simulink model "HydroPowerSheet"  (R2017b)
settings: Solver=FixedStepDiscrete  StartTime=0.0  StopTime=365  FixedStep=1  RelTol=1e-3
undefined symbols (not defined in the file or in its folder): DiscIntNeverNeededParam
settings Model: Creator=h17163  LastModifiedBy=h17163

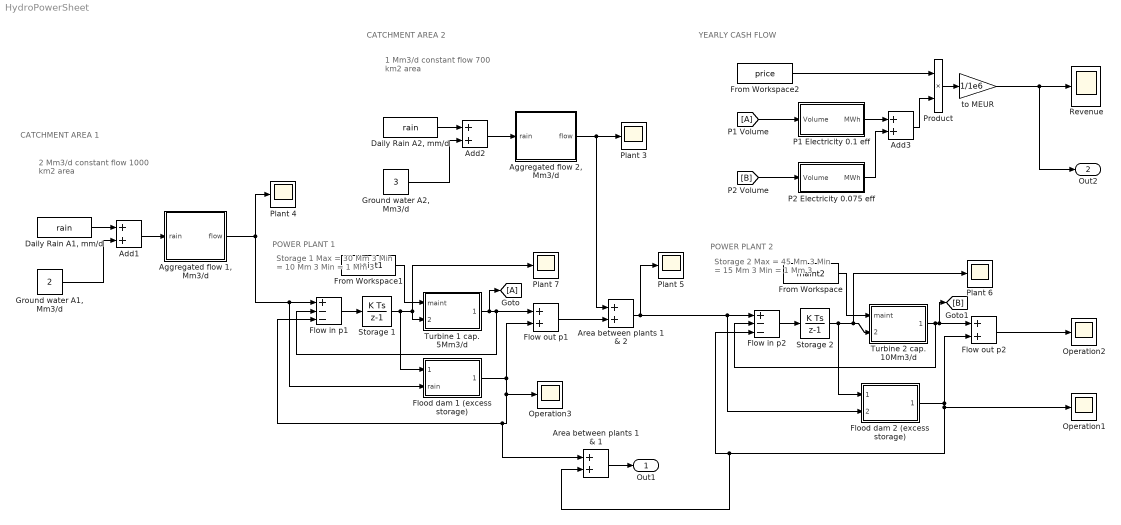
== system HydroPowerSheet ==
  note: YEARLY CASH FLOW
  note: 2 Mm3/d constant flow
      | 1000 km2 area
  note: POWER PLANT 1
  note: CATCHMENT AREA 1
  note: Storage 1
      | Max = 30 Mm 3
      | Min = 10 Mm 3
      | Min = 1 Mm 3
  note: Storage 2
      | Max = 45 Mm 3
      | Min = 15 Mm 3
      | Min = 1 Mm 3
  note: POWER PLANT 2
  note: CATCHMENT AREA 2
  note: 1 Mm3/d constant flow
      | 700 km2 area
  Add1 : Sum
  Add2 : Sum
  Add3 : Sum
  "Aggregated flow 1, Mm3/d" : MATLAB Function  TreatAsAtomicUnit=on
  "Aggregated flow 2, Mm3/d" : MATLAB Function  TreatAsAtomicUnit=on
  Area between plants 1 & 1 : Sum
  Area between plants 1 & 2 : Sum
  "Daily Rain A1, mm/d" : FromWorkspace  VariableName=rain  SampleTime=0
  "Daily Rain A2, mm/d" : FromWorkspace  VariableName=rain  SampleTime=0
  Flood dam 1 (excess storage) : MATLAB Function  TreatAsAtomicUnit=on
  Flood dam 2 (excess storage) : MATLAB Function  TreatAsAtomicUnit=on
  Flow in p1 : Sum  Inputs=+--
  Flow in p2 : Sum  Inputs=+--
  Flow out p1 : Sum
  Flow out p2 : Sum
  From Workspace : FromWorkspace  VariableName=maint2  SampleTime=0
  From Workspace1 : FromWorkspace  VariableName=maint1  SampleTime=0
  From Workspace2 : FromWorkspace  VariableName=price  SampleTime=0
  "Ground water A1, Mm3/d" : Constant  Value=2
  "Ground water A2, Mm3/d" : Constant  Value=3
  Operation1 : Scope
  Operation2 : Scope
  Operation3 : Scope
  P1 Electricity 0.1 eff : MATLAB Function  TreatAsAtomicUnit=on
  P2 Electricity 0.075 eff : MATLAB Function  TreatAsAtomicUnit=on
  Plant {3..7} (5 alike) : Scope
  Product : Product
  Revenue : Scope
  Storage 1 : DiscreteIntegrator  InitialCondition=15  InitialConditionSetting=State (most efficient)  SampleTime=-1  ICPrevOutput=DiscIntNeverNeededParam  ICPrevScaledInput=DiscIntNeverNeededParam
  Storage 2 : DiscreteIntegrator  InitialCondition=50  InitialConditionSetting=State (most efficient)  SampleTime=-1  ICPrevOutput=DiscIntNeverNeededParam  ICPrevScaledInput=DiscIntNeverNeededParam
  Turbine 1 cap. 5Mm3/d : MATLAB Function  TreatAsAtomicUnit=on
  Turbine 2 cap. 10Mm3/d : MATLAB Function  TreatAsAtomicUnit=on
  to MEUR : Gain  Gain=1/1e6
  Out1 : Outport
  Out2 : Outport  Port=2
  wires:
  Add1/1 -> "Aggregated flow 1, Mm3/d"/1(rain)
  "Aggregated flow 1, Mm3/d"/1(flow) -> Plant 4/1, Flood dam 1 (excess storage)/2(rain), Flow in p1/1
  Turbine 1 cap. 5Mm3/d/1(output) -> [A], Flow out p1/1, Flow in p1/2
  Storage 1/1 -> Plant 7/1, Turbine 1 cap. 5Mm3/d/2(storage), Flood dam 1 (excess storage)/1(storage)
  Flow in p1/1 -> Storage 1/1
  Flood dam 1 (excess storage)/1(output) -> Operation3/1, Area between plants 1 & 1/1, Flow in p1/3, Flow out p1/2
  "Daily Rain A1, mm/d"/1 -> Add1/1
  "Ground water A1, Mm3/d"/1 -> Add1/2
  Flood dam 2 (excess storage)/1(output) -> Area between plants 1 & 1/2, Flow in p2/3, Operation1/1, Flow out p2/2
  Area between plants 1 & 2/1 -> Flood dam 2 (excess storage)/2(excess), Flow in p2/1, Plant 5/1
  Flow in p2/1 -> Storage 2/1
  Turbine 2 cap. 10Mm3/d/1(output) -> [B], Flow out p2/1, Flow in p2/2
  Storage 2/1 -> Plant 6/1, Turbine 2 cap. 10Mm3/d/2(storage), Flood dam 2 (excess storage)/1(storage)
  Flow out p2/1 -> Operation2/1
  "Aggregated flow 2, Mm3/d"/1(flow) -> Area between plants 1 & 2/1, Plant 3/1
  "Ground water A2, Mm3/d"/1 -> Add2/2
  "Daily Rain A2, mm/d"/1 -> Add2/1
  Add2/1 -> "Aggregated flow 2, Mm3/d"/1(rain)
  Flow out p1/1 -> Area between plants 1 & 2/2
  Area between plants 1 & 1/1 -> Out1/1
  From Workspace/1 -> Turbine 2 cap. 10Mm3/d/1(maint)
  From Workspace1/1 -> Turbine 1 cap. 5Mm3/d/1(maint)
  [A] -> P1 Electricity 0.1 eff/1(Volume)
  P1 Electricity 0.1 eff/1(MWh) -> Add3/1
  [B] -> P2 Electricity 0.075 eff/1(Volume)
  P2 Electricity 0.075 eff/1(MWh) -> Add3/2
  Add3/1 -> Product/2
  From Workspace2/1 -> Product/1
  Product/1 -> to MEUR/1
  to MEUR/1 -> Revenue/1, Out2/1

== matlab function HydroPowerSheet/Flood dam 1 (excess storage) ==
  data: storage input; output output; rain input
function output = fcn(storage, rain)
if storage >= 30
    output = storage-30+rain;
else
    output = 0;
end

== matlab function HydroPowerSheet/Turbine 1 cap. 5Mm3//d ==
  data: maint input; storage input; output output
function output = fcn(maint, storage)
if storage > 5 & maint == 0
    output = 5;
else
    output = 0;
end

== matlab function HydroPowerSheet/Aggregated flow 1, Mm3//d ==
  data: rain input; flow output
function flow = fcn(rain)
CA1 = 1000; %Catchment area size
flow = (rain/1e3)*(CA1*1e6)/1e6;
end

== matlab function HydroPowerSheet/Flood dam 2 (excess storage) ==
  data: storage input; output output; excess input
function output = fcn(storage, excess)
if storage >= 100
    output = storage-100+excess;
else
    output = 0;
end

== matlab function HydroPowerSheet/Turbine 2 cap. 10Mm3//d ==
  data: maint input; storage input; output output
function output = fcn(maint, storage)
if storage > 10 & maint == 0
    output = 10;
else
    output = 0;
end

== matlab function HydroPowerSheet/Aggregated flow 2, Mm3//d ==
  data: rain input; flow output
function flow = fcn(rain)
CA2 = 700; %Catchment area size
flow = (rain/1e3)*(CA2*1e6)/1e6;
end

== matlab function HydroPowerSheet/P1 Electricity 0.1 eff ==
  data: Volume input; MWh output
function MWh = fcn(Volume)
% 1 ton = 1.25kWh -> 1 kton = 1.25MWh
MWh = Volume*1000*.1;
end

== matlab function HydroPowerSheet/P2 Electricity 0.075 eff ==
  data: Volume input; MWh output
function MWh = fcn(Volume)
% 1 ton = 1.25kWh -> 1 kton = 1.25MWh
MWh = Volume*1000*.075;
end
